simulink model "ArmCast_WrapV2_0"  (Simulink 8.2)
settings: Solver=FixedStepDiscrete  StartTime=0.0  StopTime=Inf  RelTol=1e-3
PreLoadFcn:
  | Ts=0.001;
  | Trajectory = load('CastingTrajectory.mat')
undefined symbols (not defined in the file or in its folder): DiscIntNeverNeededParam
libraries: simulink x15, xpclib x7, speedgoatlib_IO102 x4, speedgoatlib_IO301 x4, xpcutilitieslib x3
(part 1 of 2)
settings Model: Creator=LukePH  LastModifiedBy=LukePH  SimulationMode=external  BufferReuse=off
settings DataIOCC: SignalLoggingSaveFormat=Dataset
settings OptimizationCC: BlockReduction=off  OptimizeBlockIOStorage=off  BufferReuse=off  ExpressionFolding=off  ExpressionDepthLimit=128  LocalBlockOutputs=off
settings DebuggingCC: FcnCallInpInsideContextMsg=EnableAllAsError  StateNameClashWarn=none
settings HardwareCC: ProdIntDivRoundTo=Zero  ProdEndianess=LittleEndian  ProdHWDeviceType=Generic->32-bit x86 compatible
settings RTWCC: SystemTargetFile=xpctarget.tlc  TemplateMakefile=xpc_default_tmf  Description=xPC Target  ProcessScript=xpctarget_make_rtw_hook  RTWCompilerOptimization=On
settings xpcTargetCC: TargetFcnLib=ansi_tfl_table_tmw.mat  CodeReplacementLibrary=XPC_BLAS  ParMdlRefBuildCompliant=on  ConcurrentExecutionCompliant=on  CombineSignalStateStructs=off  MATLABClassNameForMDSCustomization=xpcAperiodicCustomization  GRTInterface=on  GenerateAllocFcn=off  xPCTaskExecutionProfile=off  xPCRL32EventNumber=5000  xPCLoadParamSetFile=off  xPCConcurrentTasks=off  xPCEnableSFAnimation=off

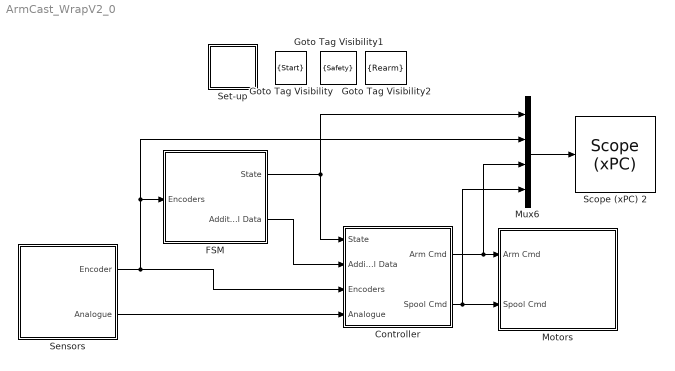
== system ArmCast_WrapV2_0 ==
  Controller : Subsystem
  FSM : Subsystem
  Goto Tag Visibility : GotoTagVisibility  GotoTag=Start
  Goto Tag Visibility1 : GotoTagVisibility  GotoTag=Safety
  Goto Tag Visibility2 : GotoTagVisibility  GotoTag=Rearm
  Motors : Subsystem
  Mux6 : Mux
  Scope (xPC) 2 : xpclib/Misc./Scope (xPC)   scopeno=10  scopetype=File  autostart=on  viewmode=Numerical  formatstr='%15.6f'  grid=on  ylimits=[-2*pi,2*pi]  nosamples=4001  noprepostsamples=0  interleave=4  triggermode=FreeRun  triggersignal=1  trigsignalfromport=off  triggerlevel=0.0  triggerslope=Either  triggerscope=1  triggersample=0  filename=data.dat  mode=Lazy  writesize=512  autorestart=on  dynamicfilemode=off  maxwritefilesize=512*1024^2
  Sensors : Subsystem
  Set-up : Subsystem
  wires:
  Sensors/1(Encoder) -> Controller/3(Encoders), FSM/1(Encoders), Mux6/2
  Sensors/2(Analogue) -> Controller/4(Analogue)
  Controller/1(Arm Cmd) -> Mux6/3, Motors/1(Arm Cmd)
  Controller/2(Spool Cmd) -> Mux6/4, Motors/2(Spool Cmd)
  FSM/1(State) -> Controller/1(State), Mux6/1
  Mux6/1 -> Scope (xPC) 2/1
  FSM/2(Additional Data) -> Controller/2(Additional Data)

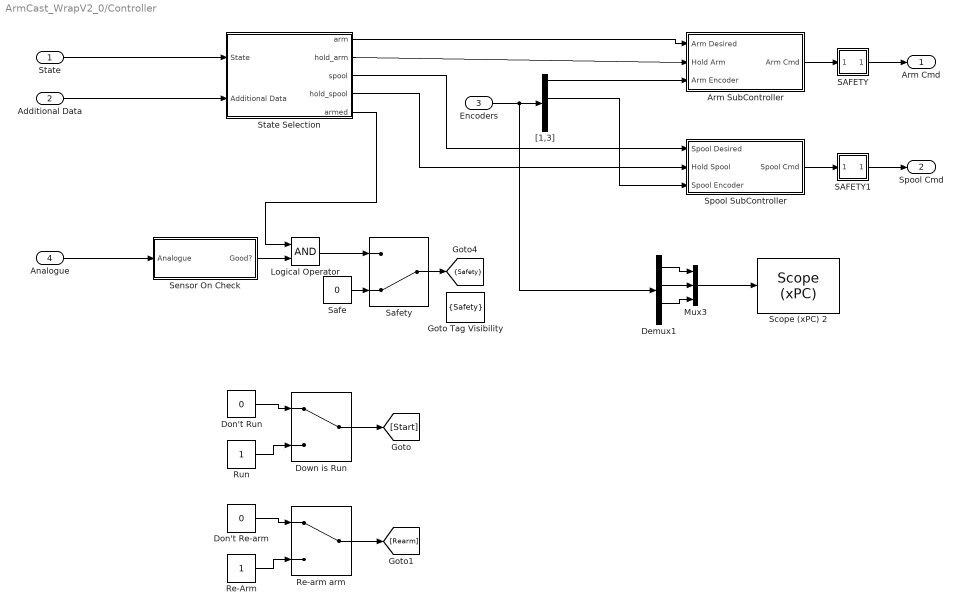
== system ArmCast_WrapV2_0/Controller ==
  State : Inport
  Additional Data : Inport  Port=2
  Encoders : Inport  Port=3
  Analogue : Inport  Port=4
  Arm SubController : Subsystem
  Demux1 : Demux  Outputs=6
  Don't Re-arm : Constant  Value=0
  Don't Run : Constant  Value=0
  Down is Run : ManualSwitch
  Goto Tag Visibility : GotoTagVisibility  GotoTag=Safety
  Logical Operator : Logic  AllPortsSameDT=off  OutDataTypeStr=boolean
  Mux3 : Mux  Inputs=3
  Re-Arm : Constant
  Re-arm arm : ManualSwitch
  Run : Constant
  SAFETY : Subsystem
  SAFETY1 : Subsystem
  Safe : Constant  Value=0
  Safety : ManualSwitch  CurrentSetting=0
  Scope (xPC) 2 : xpclib/Misc./Scope (xPC)   scopeno=4  scopetype=Target  autostart=on  viewmode=Numerical  formatstr='%15.6f'  grid=on  ylimits=[-2*pi,2*pi]  nosamples=250  noprepostsamples=0  interleave=1  triggermode=FreeRun  triggersignal=1  trigsignalfromport=off  triggerlevel=0.0  triggerslope=Either  triggerscope=1  triggersample=0  filename=data.dat  mode=Lazy  writesize=512  autorestart=off  dynamicfilemode=off  maxwritefilesize=512*1024^2
  Sensor On Check : Subsystem
  Spool SubController : Subsystem
  State Selection : Subsystem
  "[1,3]" : Demux  Outputs=6
  Arm Cmd : Outport
  Spool Cmd : Outport  Port=2
  tag scope: Safety=scoped
  wires:
  Safe/1 -> Safety/2
  Safety/1 -> [Safety]
  State Selection/5(armed) -> Logical Operator/1
  State/1 -> State Selection/1(State)
  Encoders/1 -> Demux1/1, "[1,3]"/1
  Analogue/1 -> Sensor On Check/1(Analogue)
  Logical Operator/1 -> Safety/1
  Sensor On Check/1(Good?) -> Logical Operator/2
  Additional Data/1 -> State Selection/2(Additional Data)
  Mux3/1 -> Scope (xPC) 2/1
  Demux1/1 -> Mux3/1
  Demux1/3 -> Mux3/2
  Demux1/5 -> Mux3/3
  State Selection/1(arm) -> Arm SubController/1(Arm Desired)
  "[1,3]"/1 -> Arm SubController/3(Arm Encoder)
  Arm SubController/1(Arm Cmd) -> SAFETY/1(In1)
  SAFETY/1(Out1) -> Arm Cmd/1
  Spool SubController/1(Spool Cmd) -> SAFETY1/1(In1)
  SAFETY1/1(Out1) -> Spool Cmd/1
  State Selection/3(spool) -> Spool SubController/1(Spool Desired)
  State Selection/2(hold_arm) -> Arm SubController/2(Hold Arm)
  State Selection/4(hold_spool) -> Spool SubController/2(Hold Spool)
  "[1,3]"/3 -> Spool SubController/3(Spool Encoder)
  Run/1 -> Down is Run/2
  Don't Run/1 -> Down is Run/1
  Down is Run/1 -> [Start]
  Re-Arm/1 -> Re-arm arm/2
  Don't Re-arm/1 -> Re-arm arm/1
  Re-arm arm/1 -> [Rearm]

== system ArmCast_WrapV2_0/FSM ==
  Encoders : Inport
  Clock : Clock
  Event Handler : Subsystem
  Memory1 : Memory  InheritSampleTime=on
  Switch : Switch  Criteria=u2 > Threshold
  State : Outport
  Additional Data : Outport  Port=2
  wires:
  Switch/1 -> Event Handler/2(Run Start Time), Memory1/1
  Clock/1 -> Switch/3, Event Handler/3(Clock)
  [Start] -> Switch/2, Event Handler/1(Start Signal)
  Memory1/1 -> Switch/1
  Encoders/1 -> Event Handler/4(Encoder)
  [Rearm] -> Event Handler/5(Re-arm)
  Event Handler/1(State) -> State/1
  Event Handler/2(Additional_data) -> Additional Data/1
  [Safety] -> Event Handler/6(Safety)

== system ArmCast_WrapV2_0/Motors ==
  Arm Cmd : Inport
  Spool Cmd : Inport  Port=2
  Analog output : speedgoatlib_IO102/Analog output  id=1  channels=[1,2]  range=1  ts=Ts  pciSlot=-1
  Mux4 : Mux  Inputs=2
  Scope (xPC) 4 : xpclib/Misc./Scope (xPC)   scopeno=6  scopetype=Target  autostart=on  viewmode=Numerical  formatstr='%15.6f'  grid=on  ylimits=[-2*pi,2*pi]  nosamples=250  noprepostsamples=0  interleave=1  triggermode=FreeRun  triggersignal=1  trigsignalfromport=off  triggerlevel=0.0  triggerslope=Either  triggerscope=1  triggersample=0  filename=data.dat  mode=Lazy  writesize=512  autorestart=off  dynamicfilemode=off  maxwritefilesize=512*1024^2
  wires:
  Spool Cmd/1 -> Mux4/2, Analog output/2
  Arm Cmd/1 -> Mux4/1, Analog output/1
  Mux4/1 -> Scope (xPC) 4/1

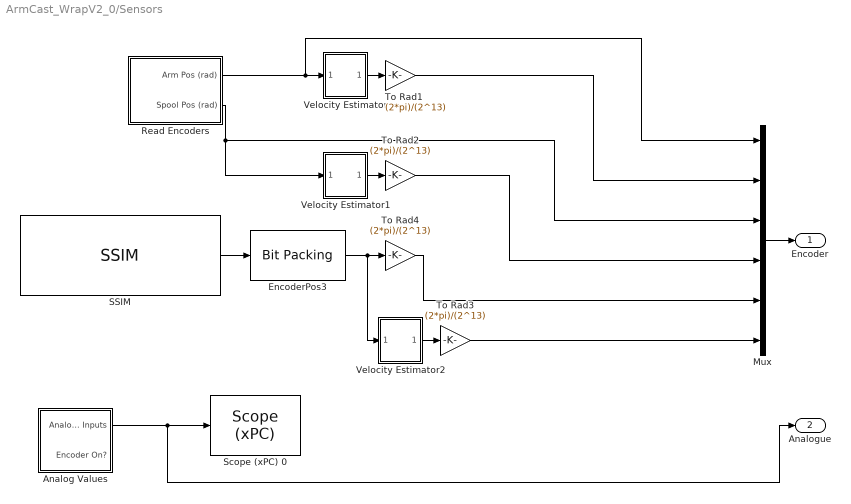
== system ArmCast_WrapV2_0/Sensors ==
  Analog Values : Subsystem
  EncoderPos3 : xpcutilitieslib/Bit Packing   MaskBitPatterns={[0:12]}  MaskPackDataType=int32  MaskPackDataSize=[1]
  Mux : Mux  Inputs=6
  Read Encoders : Subsystem
  SSIM : speedgoatlib_IO301/SSI/SSIM  id=1  chan=[3]  coding=Binary  clockDivider=[200]  wordSize=[13]  TL=[0]  TP=[990]  ssiminv=off  ts=Ts  pciSlot=-1
  "Scope (xPC) 0 " : xpclib/Misc./Scope (xPC)   scopeno=1  scopetype=Target  autostart=on  viewmode=Numerical  formatstr='%15.6f'  grid=on  ylimits=[0,0]  nosamples=250  noprepostsamples=0  interleave=1  triggermode=FreeRun  triggersignal=1  trigsignalfromport=off  triggerlevel=0.0  triggerslope=Either  triggerscope=1  triggersample=0  filename=data.dat  mode=Lazy  writesize=512  autorestart=off  dynamicfilemode=off  maxwritefilesize=512*1024^2
  To Rad{1..4} (4 alike) : Gain  Gain=(2*pi)/(2^13)  OutDataTypeStr=double
  Velocity Estimator : Subsystem  mask{SampleTime=Ts}
      mask prompts: SampleTime "Sample time (-1 for inherited):"
      mask help:
      | This Block takes in encoder values at a rate of 1 sample per Ts seconds and
      | produces an estimate of the velocity at the given time.
      mask TypeOptions SampleTime: Velocity /SystemSampleTime | Weight Calc/SystemSampleTime | Weighted Average/SystemSampleTime | Velocity /Time Constant/Value | Discrete-Time Integrator/SampleTime | Dead Zone/SampleTime | Weight Calc/9000 rad//sec^2 Cut-off/SampleTime | Weight Calc/Discrete Low Pass1/SampleTime | Weight Calc/Discrete Transfer Fcn/SampleTime | Weight Calc/Discrete Transfer Fcn1/SampleTime | Discrete Low Pass2/SampleTime | Velocity /My Difference/Delay/SampleTime | Velocity /My Difference/Sum/SampleTime
      mask Display:
      | port_label('output', 1, '')
      | port_label('input', 1, '')
  Velocity Estimator1 : Subsystem  mask{SampleTime=Ts}
      mask prompts: SampleTime "Sample time (-1 for inherited):"
      mask help:
      | This Block takes in encoder values at a rate of 1 sample per Ts seconds and
      | produces an estimate of the velocity at the given time.
      mask TypeOptions SampleTime: Velocity /SystemSampleTime | Weight Calc/SystemSampleTime | Weighted Average/SystemSampleTime | Velocity /Time Constant/Value | Discrete-Time Integrator/SampleTime | Dead Zone/SampleTime | Weight Calc/9000 rad//sec^2 Cut-off/SampleTime | Weight Calc/Discrete Low Pass1/SampleTime | Weight Calc/Discrete Transfer Fcn/SampleTime | Weight Calc/Discrete Transfer Fcn1/SampleTime | Discrete Low Pass2/SampleTime | Velocity /My Difference/Delay/SampleTime | Velocity /My Difference/Sum/SampleTime
      mask Display:
      | port_label('output', 1, '')
      | port_label('input', 1, '')
  Velocity Estimator2 : Subsystem  mask{SampleTime=Ts}
      mask prompts: SampleTime "Sample time (-1 for inherited):"
      mask help:
      | This Block takes in encoder values at a rate of 1 sample per Ts seconds and
      | produces an estimate of the velocity at the given time.
      mask TypeOptions SampleTime: Velocity /SystemSampleTime | Weight Calc/SystemSampleTime | Weighted Average/SystemSampleTime | Velocity /Time Constant/Value | Discrete-Time Integrator/SampleTime | Dead Zone/SampleTime | Weight Calc/9000 rad//sec^2 Cut-off/SampleTime | Weight Calc/Discrete Low Pass1/SampleTime | Weight Calc/Discrete Transfer Fcn/SampleTime | Weight Calc/Discrete Transfer Fcn1/SampleTime | Discrete Low Pass2/SampleTime | Velocity /My Difference/Delay/SampleTime | Velocity /My Difference/Sum/SampleTime
      mask Display:
      | port_label('output', 1, '')
      | port_label('input', 1, '')
  Encoder : Outport
  Analogue : Outport  Port=2
  wires:
  Velocity Estimator1/1(Out1) -> To Rad2/1
  To Rad1/1 -> Mux/2
  Velocity Estimator/1(Out1) -> To Rad1/1
  Read Encoders/1(Arm Pos (rad)) -> Velocity Estimator/1(In1), Mux/1
  Read Encoders/2(Spool Pos (rad)) -> Velocity Estimator1/1(In1), Mux/3
  SSIM/1 -> EncoderPos3/1
  EncoderPos3/1 -> Velocity Estimator2/1(In1), To Rad4/1
  Velocity Estimator2/1(Out1) -> To Rad3/1
  Mux/1 -> Encoder/1
  To Rad4/1 -> Mux/5
  To Rad3/1 -> Mux/6
  To Rad2/1 -> Mux/4
  Analog Values/1(Analog Inputs) -> Analogue/1, "Scope (xPC) 0 "/1

== system ArmCast_WrapV2_0/Set-up ==
  AnalogSetUp : Subsystem
  Digital output : speedgoatlib_IO301/DIO/Digital output  id=1  channelGroup=Lower  portType=32 ports of type double  lowerDirection=[0,0,0,0,0,0,1,1,1,1,1,1,1,1,1,1]  upperDirection=[1,1,1,1,1,1,1,1,0,0,0,0,0,0,0,0]  ts=Ts  pciSlot=-1
  Disable NST : Constant  Value=0
  Do Not Zero Arm : Constant
  Do Not Zero Spool : Constant
  Setup : speedgoatlib_IO301/Setup/Setup  group=Lower channel group setup  id=1  fpga1=speedgoat_IO301_CI_01230  pciSlot=-1  lowerDirection=[0,0,0,0,0,0,1,1,1,1,1,1,1,1,1,1]  lowerReset=[1]  lowerValue=[1]  upperDirection=[1, 1, 1, 1, 1, 1, 1, 1, 0, 0, 0, 0, 0, 0, 0, 0]  upperReset=[1]  upperValue=[0]
  wires:
  Disable NST/1 -> Digital output/19, Digital output/17
  Do Not Zero Arm/1 -> Digital output/18
  Do Not Zero Spool/1 -> Digital output/20

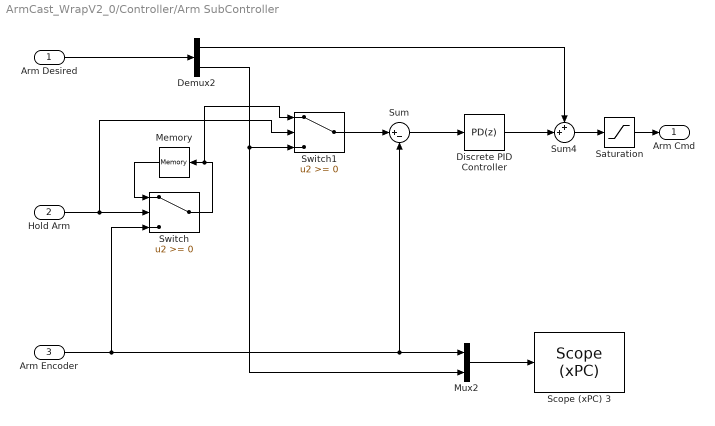
== system ArmCast_WrapV2_0/Controller/Arm SubController ==
  Arm Desired : Inport
  Hold Arm : Inport  Port=2
  Arm Encoder : Inport  Port=3
  Demux2 : Demux  Outputs=2
  Discrete PID Controller : simulink/Continuous/PID Controller  Controller=PD  TimeDomain=Discrete-time  SampleTime=Ts  IntegratorMethod=Forward Euler  FilterMethod=Forward Euler  Form=Parallel  P=30  I=0  D=.15  N=100  InitialConditionSource=internal  InitialConditionForIntegrator=0  InitialConditionForFilter=0  ExternalReset=none  LimitOutput=on  UpperSaturationLimit=6  LowerSaturationLimit=-6  LinearizeAsGain=off  AntiWindupMode=clamping  Kb=1  TrackingMode=off  Kt=1  PParamMin=[]  PParamMax=[]  IParamMin=[]  IParamMax=[]  DParamMin=[]  DParamMax=[]  NParamMin=[]  NParamMax=[]  KbParamMin=[]  KbParamMax=[]  KtParamMin=[]  KtParamMax=[]  POutMin=[]  POutMax=[]  IOutMin=[]  IOutMax=[]  DOutMin=[]  DOutMax=[]  NOutMin=[]  NOutMax=[]  KbOutMin=[]  KbOutMax=[]  KtOutMin=[]  KtOutMax=[]  IntegratorOutMin=[]  IntegratorOutMax=[]  FilterOutMin=[]  FilterOutMax=[]  SumOutMin=[]  SumOutMax=[]  SumI1OutMin=[]  SumI1OutMax=[]  SumI2OutMin=[]  SumI2OutMax=[]  SumI3OutMin=[]  SumI3OutMax=[]  SumDOutMin=[]  SumDOutMax=[]  SaturationOutMin=[]  SaturationOutMax=[]  IntegratorContinuousStateAttributes=''  IntegratorStateMustResolveToSignalObject=off  IntegratorRTWStateStorageClass=Auto  FilterContinuousStateAttributes=''  FilterStateMustResolveToSignalObject=off  FilterRTWStateStorageClass=Auto
  Memory : Memory
  Mux2 : Mux  Inputs=2
  Saturation : Saturate  UpperLimit=6  LowerLimit=-6
  Scope (xPC) 3 : xpclib/Misc./Scope (xPC)   scopeno=2  scopetype=Target  autostart=on  viewmode=Graphical redraw  formatstr='%15.6f'  grid=on  ylimits=[-2*pi,2*pi]  nosamples=250  noprepostsamples=0  interleave=1  triggermode=FreeRun  triggersignal=1  trigsignalfromport=off  triggerlevel=0.0  triggerslope=Either  triggerscope=1  triggersample=0  filename=data.dat  mode=Lazy  writesize=512  autorestart=off  dynamicfilemode=off  maxwritefilesize=512*1024^2
  Sum : Sum  Inputs=|+-
  Sum4 : Sum  Inputs=++|
  Switch : Switch
  Switch1 : Switch
  Arm Cmd : Outport
  wires:
  Mux2/1 -> Scope (xPC) 3/1
  Arm Desired/1 -> Demux2/1
  Sum/1 -> Discrete PID Controller/1
  Saturation/1 -> Arm Cmd/1
  Discrete PID Controller/1 -> Sum4/2
  Sum4/1 -> Saturation/1
  Arm Encoder/1 -> Sum/2, Mux2/1, Switch/3
  Demux2/1 -> Sum4/1
  Demux2/2 -> Switch1/3, Mux2/2
  Switch/1 -> Switch1/1, Memory/1
  Memory/1 -> Switch/1
  Hold Arm/1 -> Switch/2, Switch1/2
  Switch1/1 -> Sum/1

== system ArmCast_WrapV2_0/Controller/SAFETY ==
  In1 : Inport
  Null Cmd2 : Constant  Value=0
  Switch : Switch  Criteria=u2 > Threshold
  Out1 : Outport
  wires:
  Switch/1 -> Out1/1
  Null Cmd2/1 -> Switch/3
  [Safety] -> Switch/2
  In1/1 -> Switch/1

== system ArmCast_WrapV2_0/Controller/SAFETY1 ==
  In1 : Inport
  Null Cmd2 : Constant  Value=0
  Switch : Switch  Criteria=u2 > Threshold
  Out1 : Outport
  wires:
  In1/1 -> Switch/1
  [Safety] -> Switch/2
  Null Cmd2/1 -> Switch/3
  Switch/1 -> Out1/1

== system ArmCast_WrapV2_0/Controller/Sensor On Check ==
  Analogue : Inport
  Constant : Constant  Value=3.25
  Demux1 : Demux
  Relational Operator : RelationalOperator  Operator=>  OutDataTypeStr=fixdt(1,16)
  Good? : Outport
  wires:
  Relational Operator/1 -> Good?/1
  Demux1/4 -> Relational Operator/1
  Constant/1 -> Relational Operator/2
  Analogue/1 -> Demux1/1

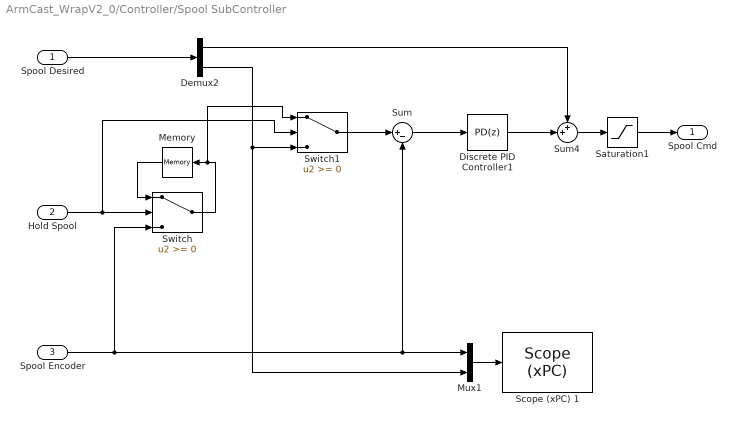
== system ArmCast_WrapV2_0/Controller/Spool SubController ==
  Spool Desired : Inport
  Hold Spool : Inport  Port=2
  Spool Encoder : Inport  Port=3
  Demux2 : Demux  Outputs=2
  Discrete PID Controller1 : simulink/Continuous/PID Controller  Controller=PD  TimeDomain=Discrete-time  SampleTime=Ts  IntegratorMethod=Forward Euler  FilterMethod=Forward Euler  Form=Parallel  P=20  I=0  D=.05  N=100  InitialConditionSource=internal  InitialConditionForIntegrator=0  InitialConditionForFilter=0  ExternalReset=none  LimitOutput=on  UpperSaturationLimit=6  LowerSaturationLimit=-6  LinearizeAsGain=off  AntiWindupMode=clamping  Kb=1  TrackingMode=off  Kt=1  PParamMin=[]  PParamMax=[]  IParamMin=[]  IParamMax=[]  DParamMin=[]  DParamMax=[]  NParamMin=[]  NParamMax=[]  KbParamMin=[]  KbParamMax=[]  KtParamMin=[]  KtParamMax=[]  POutMin=[]  POutMax=[]  IOutMin=[]  IOutMax=[]  DOutMin=[]  DOutMax=[]  NOutMin=[]  NOutMax=[]  KbOutMin=[]  KbOutMax=[]  KtOutMin=[]  KtOutMax=[]  IntegratorOutMin=[]  IntegratorOutMax=[]  FilterOutMin=[]  FilterOutMax=[]  SumOutMin=[]  SumOutMax=[]  SumI1OutMin=[]  SumI1OutMax=[]  SumI2OutMin=[]  SumI2OutMax=[]  SumI3OutMin=[]  SumI3OutMax=[]  SumDOutMin=[]  SumDOutMax=[]  SaturationOutMin=[]  SaturationOutMax=[]  IntegratorContinuousStateAttributes=''  IntegratorStateMustResolveToSignalObject=off  IntegratorRTWStateStorageClass=Auto  FilterContinuousStateAttributes=''  FilterStateMustResolveToSignalObject=off  FilterRTWStateStorageClass=Auto
  Memory : Memory
  Mux1 : Mux  Inputs=2
  Saturation1 : Saturate  UpperLimit=6  LowerLimit=-6
  Scope (xPC) 1 : xpclib/Misc./Scope (xPC)   scopeno=3  scopetype=Target  autostart=on  viewmode=Graphical redraw  formatstr='%15.6f'  grid=on  ylimits=[-2*pi,2*pi]  nosamples=250  noprepostsamples=0  interleave=1  triggermode=FreeRun  triggersignal=1  trigsignalfromport=off  triggerlevel=0.0  triggerslope=Either  triggerscope=1  triggersample=0  filename=data.dat  mode=Lazy  writesize=512  autorestart=off  dynamicfilemode=off  maxwritefilesize=512*1024^2
  Sum : Sum  Inputs=|+-
  Sum4 : Sum  Inputs=++|
  Switch : Switch
  Switch1 : Switch
  Spool Cmd : Outport
  wires:
  Mux1/1 -> Scope (xPC) 1/1
  Saturation1/1 -> Spool Cmd/1
  Spool Desired/1 -> Demux2/1
  Spool Encoder/1 -> Sum/2, Mux1/1, Switch/3
  Demux2/2 -> Switch1/3, Mux1/2
  Switch/1 -> Switch1/1, Memory/1
  Memory/1 -> Switch/1
  Hold Spool/1 -> Switch/2, Switch1/2
  Switch1/1 -> Sum/1
  Sum4/1 -> Saturation1/1
  Discrete PID Controller1/1 -> Sum4/2
  Sum/1 -> Discrete PID Controller1/1
  Demux2/1 -> Sum4/1

== system ArmCast_WrapV2_0/Controller/State Selection ==
  State : Inport
  Additional Data : Inport  Port=2
  Clock2 : Clock
      settings: Decimation=5
  MATLAB Function : MATLAB Function  TreatAsAtomicUnit=on
  Mux : Mux  Inputs=2
  Mux1 : Mux  Inputs=2
  arm : Outport
  hold_arm : Outport  Port=2
  spool : Outport  Port=3
  hold_spool : Outport  Port=4
  armed : Outport  Port=5
  wires:
  Clock2/1 -> MATLAB Function/3(time)
  State/1 -> MATLAB Function/1(state)
  MATLAB Function/7(armed) -> armed/1
  Additional Data/1 -> MATLAB Function/2(additional_data)
  MATLAB Function/3(hold_arm) -> hold_arm/1
  MATLAB Function/6(hold_spool) -> hold_spool/1
  MATLAB Function/1(ud_ar) -> Mux/1
  MATLAB Function/2(xd_ar) -> Mux/2
  Mux/1 -> arm/1
  MATLAB Function/4(ud_sp) -> Mux1/1
  MATLAB Function/5(xd_sp) -> Mux1/2
  Mux1/1 -> spool/1

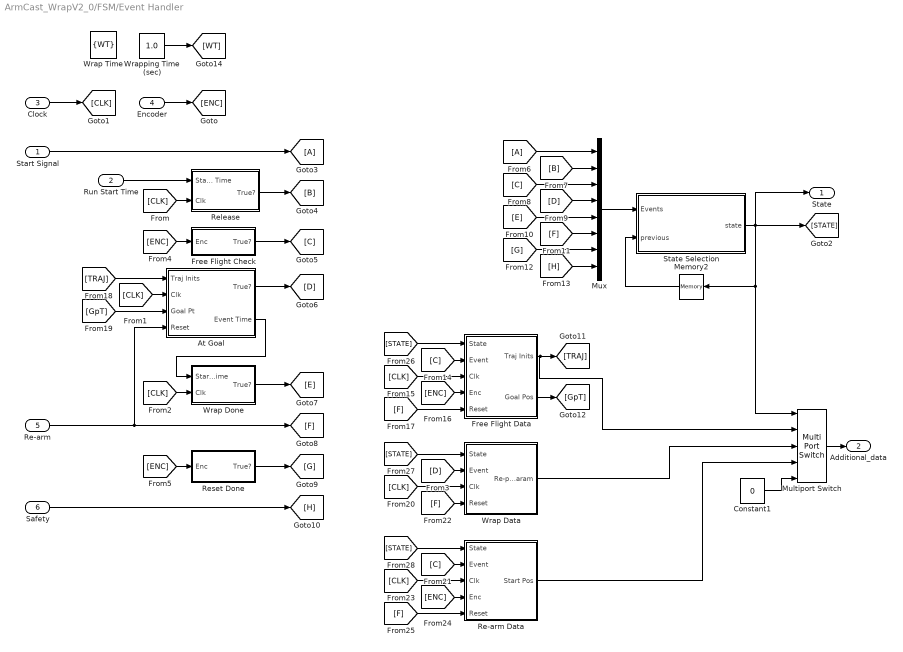
== system ArmCast_WrapV2_0/FSM/Event Handler ==
  Start Signal : Inport
  Run Start Time : Inport  Port=2
  Clock : Inport  Port=3
  Encoder : Inport  Port=4
  Re-arm : Inport  Port=5
  Safety : Inport  Port=6
  At Goal : Subsystem
  Constant1 : Constant  Value=0
  Free Flight Check : Subsystem
  Free Flight Data : Subsystem
  Memory2 : Memory
  Multiport Switch : MultiPortSwitch  Inputs=4
  Mux : Mux  Inputs=8
  Re-arm Data : Subsystem
  Release : Subsystem
  Reset Done : Subsystem
  State Selection : MATLAB Function  TreatAsAtomicUnit=on
  Wrap Data : Subsystem
  Wrap Done : Subsystem
  Wrap Time : GotoTagVisibility  GotoTag=WT
  Wrapping Time (sec) : Constant  Value=1.0
  State : Outport
  Additional_data : Outport  Port=2
  wires:
  Re-arm/1 -> At Goal/4(Reset), [F]
  Run Start Time/1 -> Release/1(Start Time)
  Encoder/1 -> [ENC]
  Clock/1 -> [CLK]
  [CLK] -> Release/2(Clk)
  [CLK] -> At Goal/2(Clk)
  [CLK] -> Wrap Done/2(Clk)
  [ENC] -> Free Flight Check/1(Enc)
  [ENC] -> Reset Done/1(Enc)
  Start Signal/1 -> [A]
  Release/1(True?) -> [B]
  Free Flight Check/1(True?) -> [C]
  At Goal/1(True?) -> [D]
  Wrap Done/1(True?) -> [E]
  Reset Done/1(True?) -> [G]
  Safety/1 -> [H]
  [B] -> Mux/2
  [F] -> Mux/6
  [D] -> Mux/4
  [H] -> Mux/8
  [C] -> Mux/3
  [E] -> Mux/5
  [A] -> Mux/1
  [G] -> Mux/7
  [C] -> Free Flight Data/2(Event)
  [CLK] -> Free Flight Data/3(Clk)
  [ENC] -> Free Flight Data/4(Enc)
  [F] -> Free Flight Data/5(Reset)
  [TRAJ] -> At Goal/1(Traj Inits)
  Free Flight Data/2(Goal Pos) -> [GpT]
  [GpT] -> At Goal/3(Goal Pt)
  At Goal/2(Event Time) -> Wrap Done/1(Start Time)
  [CLK] -> Wrap Data/3(Clk)
  [F] -> Wrap Data/4(Reset)
  Wrap Data/1(Re-pos Param) -> Multiport Switch/3
  Multiport Switch/1 -> Additional_data/1
  Free Flight Data/1(Traj Inits) -> Multiport Switch/2, [TRAJ]
  Wrapping Time (sec)/1 -> [WT]
  [CLK] -> Re-arm Data/3(Clk)
  [ENC] -> Re-arm Data/4(Enc)
  [F] -> Re-arm Data/5(Reset)
  Re-arm Data/1(Start Pos) -> Multiport Switch/4
  Constant1/1 -> Multiport Switch/5
  Mux/1 -> State Selection/1(Events)
  Memory2/1 -> State Selection/2(previous)
  [STATE] -> Free Flight Data/1(State)
  [D] -> Wrap Data/2(Event)
  [STATE] -> Wrap Data/1(State)
  [C] -> Re-arm Data/2(Event)
  [STATE] -> Re-arm Data/1(State)
  State Selection/1(state) -> State/1, [STATE], Multiport Switch/1, Memory2/1

== system ArmCast_WrapV2_0/Sensors/Analog Values ==
  Analog input : speedgoatlib_IO102/Analog input  id=1  channels=[1,2,3,4]  range=1  high_voltage=off  adCoupling=2  ts=Ts  pciSlot=-1
  Constant : Constant  Value=3.25
  Mux : Mux
  Relational Operator : RelationalOperator  Operator=>  OutDataTypeStr=fixdt(1,16)
  Analog Inputs : Outport
  Encoder On? : Outport  Port=2
  wires:
  Mux/1 -> Analog Inputs/1
  Relational Operator/1 -> Encoder On?/1
  Constant/1 -> Relational Operator/2
  Analog input/1 -> Mux/1
  Analog input/2 -> Mux/2
  Analog input/3 -> Mux/3
  Analog input/4 -> Relational Operator/1, Mux/4

== system ArmCast_WrapV2_0/Sensors/Read Encoders ==
  EncoderPos : xpcutilitieslib/Bit Packing   MaskBitPatterns={[0:16]}  MaskPackDataType=int32  MaskPackDataSize=[1]
  EncoderPos1 : xpcutilitieslib/Bit Packing   MaskBitPatterns={[0:16]}  MaskPackDataType=int32  MaskPackDataSize=[1]
  SSIM : speedgoatlib_IO301/SSI/SSIM  id=1  chan=[1:2]  coding=Gray  clockDivider=[200]  wordSize=[17]  TL=[0]  TP=[990]  ssiminv=off  ts=Ts  pciSlot=-1
  Spike Removal : Subsystem
  To Rad : Gain  Gain=(2*pi)/(2^17)  OutDataTypeStr=double
  To Rad1 : Gain  Gain=-(2*pi)/(2^17)  OutDataTypeStr=double
  Wrap Encoder Values : Subsystem
  Arm Pos (rad) : Outport
  Spool Pos (rad) : Outport  Port=2
  wires:
  Wrap Encoder Values/1(Wrapped Values) -> Spike Removal/1(Encoder)
  EncoderPos1/1 -> Wrap Encoder Values/1(Raw Input)
  Spike Removal/1(Filtered) -> To Rad1/1
  To Rad1/1 -> Spool Pos (rad)/1
  SSIM/2 -> EncoderPos1/1
  To Rad/1 -> Arm Pos (rad)/1
  EncoderPos/1 -> To Rad/1
  SSIM/1 -> EncoderPos/1

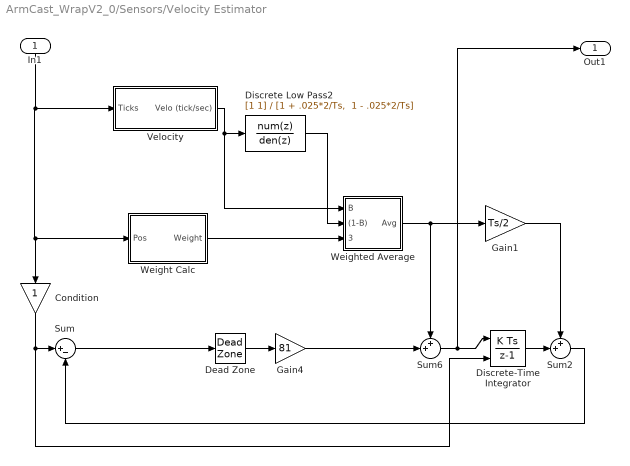
== system ArmCast_WrapV2_0/Sensors/Velocity Estimator ==
  In1 : Inport
  Condition : Gain  OutMin=0  OutMax=10^9  OutDataTypeStr=double
  Dead Zone : DeadZone  LowerValue=-1  UpperValue=1  SampleTime=SampleTime  SaturateOnIntegerOverflow=on
  Discrete Low Pass2 : DiscreteTransferFcn  Numerator=[1 1]  Denominator="[1 + .025*2/Ts,  1 - .025*2/Ts]"  SampleTime=SampleTime
  Discrete-Time Integrator : DiscreteIntegrator  InitialConditionSource=external  SampleTime=SampleTime  ICPrevOutput=DiscIntNeverNeededParam  ICPrevScaledInput=DiscIntNeverNeededParam
  Gain1 : Gain  Gain=Ts/2
  Gain4 : Gain  Gain=81
  Sum : Sum  Inputs=|+-
  Sum2 : Sum  Inputs=++|
  Sum6 : Sum  Inputs=++|
  "Velocity " : Subsystem  SystemSampleTime=SampleTime
  Weight Calc : Subsystem  SystemSampleTime=SampleTime
  Weighted Average : Subsystem  SystemSampleTime=SampleTime
  Out1 : Outport
  wires:
  Condition/1 -> Sum/1, Discrete-Time Integrator/2
  In1/1 -> "Velocity "/1(Ticks), Weight Calc/1(Pos), Condition/1
  "Velocity "/1(Velo (tick/sec)) -> Discrete Low Pass2/1, Weighted Average/1("B ")
  Sum/1 -> Dead Zone/1
  Gain4/1 -> Sum6/2
  Weighted Average/1(Avg) -> Gain1/1, Sum6/1
  Dead Zone/1 -> Gain4/1
  Sum6/1 -> Discrete-Time Integrator/1, Out1/1
  Discrete Low Pass2/1 -> Weighted Average/2((1-B))
  Sum2/1 -> Sum/2
  Discrete-Time Integrator/1 -> Sum2/2
  Gain1/1 -> Sum2/1
  Weight Calc/1(Weight) -> Weighted Average/3(Weight)

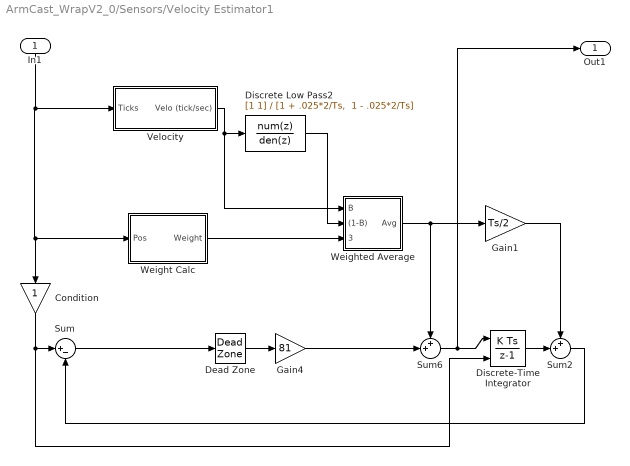
== system ArmCast_WrapV2_0/Sensors/Velocity Estimator1 ==
  In1 : Inport
  Condition : Gain  OutMin=0  OutMax=10^9  OutDataTypeStr=double
  Dead Zone : DeadZone  LowerValue=-1  UpperValue=1  SampleTime=SampleTime  SaturateOnIntegerOverflow=on
  Discrete Low Pass2 : DiscreteTransferFcn  Numerator=[1 1]  Denominator="[1 + .025*2/Ts,  1 - .025*2/Ts]"  SampleTime=SampleTime
  Discrete-Time Integrator : DiscreteIntegrator  InitialConditionSource=external  SampleTime=SampleTime  ICPrevOutput=DiscIntNeverNeededParam  ICPrevScaledInput=DiscIntNeverNeededParam
  Gain1 : Gain  Gain=Ts/2
  Gain4 : Gain  Gain=81
  Sum : Sum  Inputs=|+-
  Sum2 : Sum  Inputs=++|
  Sum6 : Sum  Inputs=++|
  "Velocity " : Subsystem  SystemSampleTime=SampleTime
  Weight Calc : Subsystem  SystemSampleTime=SampleTime
  Weighted Average : Subsystem  SystemSampleTime=SampleTime
  Out1 : Outport
  wires:
  Condition/1 -> Sum/1, Discrete-Time Integrator/2
  In1/1 -> "Velocity "/1(Ticks), Weight Calc/1(Pos), Condition/1
  "Velocity "/1(Velo (tick/sec)) -> Discrete Low Pass2/1, Weighted Average/1("B ")
  Sum/1 -> Dead Zone/1
  Gain4/1 -> Sum6/2
  Weighted Average/1(Avg) -> Gain1/1, Sum6/1
  Dead Zone/1 -> Gain4/1
  Sum6/1 -> Discrete-Time Integrator/1, Out1/1
  Discrete Low Pass2/1 -> Weighted Average/2((1-B))
  Sum2/1 -> Sum/2
  Discrete-Time Integrator/1 -> Sum2/2
  Gain1/1 -> Sum2/1
  Weight Calc/1(Weight) -> Weighted Average/3(Weight)

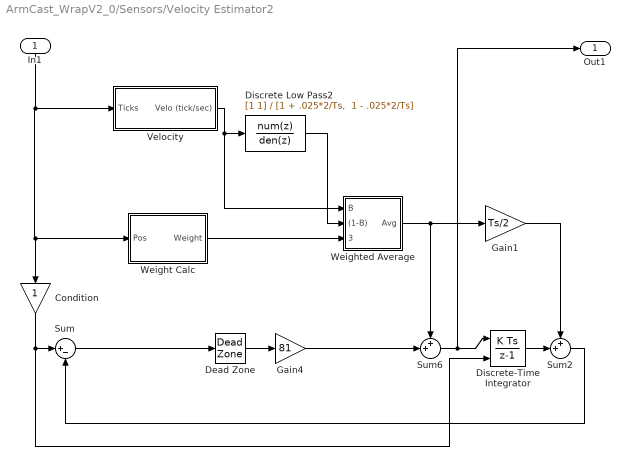
== system ArmCast_WrapV2_0/Sensors/Velocity Estimator2 ==
  In1 : Inport
  Condition : Gain  OutMin=0  OutMax=10^9  OutDataTypeStr=double
  Dead Zone : DeadZone  LowerValue=-1  UpperValue=1  SampleTime=SampleTime  SaturateOnIntegerOverflow=on
  Discrete Low Pass2 : DiscreteTransferFcn  Numerator=[1 1]  Denominator="[1 + .025*2/Ts,  1 - .025*2/Ts]"  SampleTime=SampleTime
  Discrete-Time Integrator : DiscreteIntegrator  InitialConditionSource=external  SampleTime=SampleTime  ICPrevOutput=DiscIntNeverNeededParam  ICPrevScaledInput=DiscIntNeverNeededParam
  Gain1 : Gain  Gain=Ts/2
  Gain4 : Gain  Gain=81
  Sum : Sum  Inputs=|+-
  Sum2 : Sum  Inputs=++|
  Sum6 : Sum  Inputs=++|
  "Velocity " : Subsystem  SystemSampleTime=SampleTime
  Weight Calc : Subsystem  SystemSampleTime=SampleTime
  Weighted Average : Subsystem  SystemSampleTime=SampleTime
  Out1 : Outport
  wires:
  Weight Calc/1(Weight) -> Weighted Average/3(Weight)
  Gain1/1 -> Sum2/1
  Discrete-Time Integrator/1 -> Sum2/2
  Sum2/1 -> Sum/2
  Discrete Low Pass2/1 -> Weighted Average/2((1-B))
  Sum6/1 -> Out1/1, Discrete-Time Integrator/1
  Dead Zone/1 -> Gain4/1
  Weighted Average/1(Avg) -> Sum6/1, Gain1/1
  Gain4/1 -> Sum6/2
  Sum/1 -> Dead Zone/1
  "Velocity "/1(Velo (tick/sec)) -> Weighted Average/1("B "), Discrete Low Pass2/1
  In1/1 -> Condition/1, Weight Calc/1(Pos), "Velocity "/1(Ticks)
  Condition/1 -> Discrete-Time Integrator/2, Sum/1

== system ArmCast_WrapV2_0/Set-up/AnalogSetUp ==
  Analog input : speedgoatlib_IO102/Analog input  Commented=on  id=1  channels=[1,2]  range=1  high_voltage=off  adCoupling=1  ts=Ts  pciSlot=-1
  Mux : Mux  Commented=on  Inputs=2
  Scope (xPC) 1 : xpclib/Misc./Scope (xPC)   Commented=on  scopeno=4  scopetype=Target  autostart=on  viewmode=Graphical redraw  formatstr='%15.6f'  grid=on  ylimits=[0,0]  nosamples=250  noprepostsamples=0  interleave=1  triggermode=FreeRun  triggersignal=1  trigsignalfromport=off  triggerlevel=0.0  triggerslope=Either  triggerscope=1  triggersample=0  filename=data.dat  mode=Lazy  writesize=512  autorestart=off  dynamicfilemode=off  maxwritefilesize=512*1024^2
  SetupAnalog : speedgoatlib_IO102/Setup  group=Analog input setup  id=1  range=+-10V  cal=off  pciSlot=-1  adChannelMode=Multiple-channel (enter number of channels below)  adChannel=4  adCoupling=Single-ended  daChannel=[1,2]  daReset=[1,1]  daInitValue=[0,0]  diChannel=[1]  doChannel=[1]  doReset=[1]  doInitValue=[0]
  wires:
  Mux/1 -> Scope (xPC) 1/1
  Analog input/1 -> Mux/1
  Analog input/2 -> Mux/2

== system ArmCast_WrapV2_0/FSM/Event Handler/At Goal ==
  Traj Inits : Inport
  Clk : Inport  Port=2
  Goal Pt : Inport  Port=3
  Reset : Inport  Port=4
  Latching Switch1 : Subsystem
  MATLAB Function : MATLAB Function  TreatAsAtomicUnit=on
  Memory2 : Memory  X0=false
  True? : Outport
  Event Time : Outport  Port=2
  wires:
  Memory2/1 -> Latching Switch1/2(If True)
  Latching Switch1/1(Out) -> Event Time/1, Memory2/1
  Clk/1 -> MATLAB Function/1(time), Latching Switch1/3(If False)
  Reset/1 -> Latching Switch1/4(Reset)
  Goal Pt/1 -> MATLAB Function/2(goal_pos)
  Traj Inits/1 -> MATLAB Function/3(trajectory_data)
  MATLAB Function/1(True) -> True?/1, Latching Switch1/1(T/F)

== system ArmCast_WrapV2_0/FSM/Event Handler/Free Flight Check ==
  Enc : Inport
  Add : Sum  Inputs=+-
  Compare To Zero : simulink/Logic and Bit Operations/Compare To Zero  relop=>=  OutDataTypeStr=boolean
  Compare To Zero1 : simulink/Logic and Bit Operations/Compare To Zero  relop=>  OutDataTypeStr=boolean
  Demux : Demux  Outputs=6
  Logical Operator : Logic  AllPortsSameDT=off  OutDataTypeStr=boolean
  Memory : Memory
  True? : Outport
  wires:
  Enc/1 -> Demux/1
  Memory/1 -> Add/2
  Add/1 -> Compare To Zero/1
  Compare To Zero1/1 -> Logical Operator/1
  Compare To Zero/1 -> Logical Operator/2
  Logical Operator/1 -> True?/1
  Demux/6 -> Compare To Zero1/1, Add/1, Memory/1

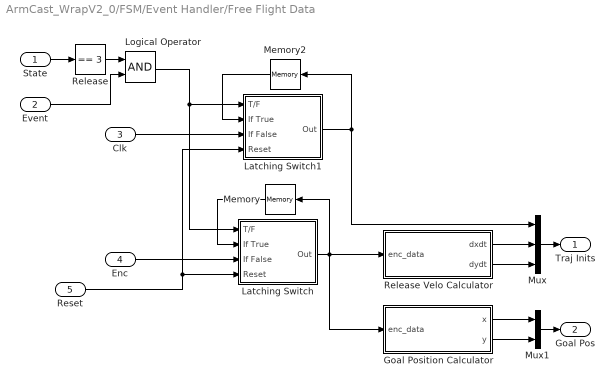
== system ArmCast_WrapV2_0/FSM/Event Handler/Free Flight Data ==
  State : Inport
  Event : Inport  Port=2
  Clk : Inport  Port=3
  Enc : Inport  Port=4
  Reset : Inport  Port=5
  Goal Position Calculator : MATLAB Function  TreatAsAtomicUnit=on
  Latching Switch : Subsystem
  Latching Switch1 : Subsystem
  Logical Operator : Logic  AllPortsSameDT=off  OutDataTypeStr=boolean
  Memory : Memory  X0=false
  Memory2 : Memory  X0=false
  Mux : Mux  Inputs=3
  Mux1 : Mux  Inputs=2
  Release : simulink/Logic and Bit Operations/Compare To Constant  relop===  const=3  OutDataTypeStr=boolean
  Release Velo Calculator : MATLAB Function  TreatAsAtomicUnit=on
  Traj Inits : Outport
  Goal Pos : Outport  Port=2
  wires:
  Event/1 -> Logical Operator/2
  Latching Switch/1(Out) -> Goal Position Calculator/1(enc_data), Memory/1, Release Velo Calculator/1(enc_data)
  Memory/1 -> Latching Switch/2(If True)
  Release Velo Calculator/1(dxdt) -> Mux/2
  Release Velo Calculator/2(dydt) -> Mux/3
  Latching Switch1/1(Out) -> Memory2/1, Mux/1
  Reset/1 -> Latching Switch1/4(Reset), Latching Switch/4(Reset)
  Memory2/1 -> Latching Switch1/2(If True)
  Clk/1 -> Latching Switch1/3(If False)
  Mux/1 -> Traj Inits/1
  Enc/1 -> Latching Switch/3(If False)
  Goal Position Calculator/2(y) -> Mux1/2
  Goal Position Calculator/1(x) -> Mux1/1
  Mux1/1 -> Goal Pos/1
  State/1 -> Release/1
  Release/1 -> Logical Operator/1
  Logical Operator/1 -> Latching Switch/1(T/F), Latching Switch1/1(T/F)

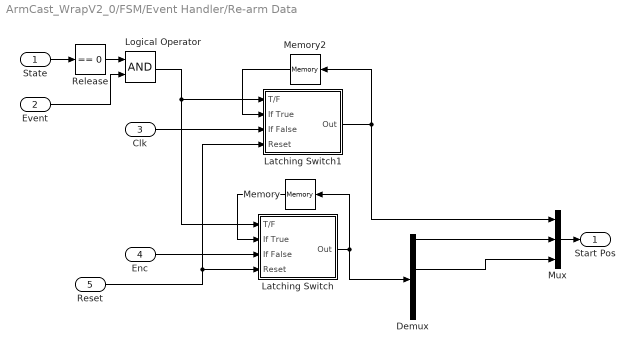
== system ArmCast_WrapV2_0/FSM/Event Handler/Re-arm Data ==
  State : Inport
  Event : Inport  Port=2
  Clk : Inport  Port=3
  Enc : Inport  Port=4
  Reset : Inport  Port=5
  Demux : Demux  Outputs=6
  Latching Switch : Subsystem
  Latching Switch1 : Subsystem
  Logical Operator : Logic  AllPortsSameDT=off  OutDataTypeStr=boolean
  Memory : Memory  X0=false
  Memory2 : Memory  X0=false
  Mux : Mux  Inputs=3
  Release : simulink/Logic and Bit Operations/Compare To Constant  relop===  const=0  OutDataTypeStr=boolean
  Start Pos : Outport
  wires:
  Enc/1 -> Latching Switch/3(If False)
  Mux/1 -> Start Pos/1
  Clk/1 -> Latching Switch1/3(If False)
  Memory2/1 -> Latching Switch1/2(If True)
  Reset/1 -> Latching Switch/4(Reset), Latching Switch1/4(Reset)
  Latching Switch1/1(Out) -> Mux/1, Memory2/1
  Memory/1 -> Latching Switch/2(If True)
  Latching Switch/1(Out) -> Memory/1, Demux/1
  Logical Operator/1 -> Latching Switch/1(T/F), Latching Switch1/1(T/F)
  Demux/1 -> Mux/2
  Demux/3 -> Mux/3
  Event/1 -> Logical Operator/2
  State/1 -> Release/1
  Release/1 -> Logical Operator/1

== system ArmCast_WrapV2_0/FSM/Event Handler/Release ==
  Start Time : Inport
  Clk : Inport  Port=2
  Add1 : Sum  Inputs=+-
  Relational Operator : RelationalOperator  OutDataTypeStr=boolean
  Release Time : Constant  Value=2.6
  True? : Outport
  wires:
  Start Time/1 -> Add1/2
  Relational Operator/1 -> True?/1
  Clk/1 -> Add1/1
  Release Time/1 -> Relational Operator/2
  Add1/1 -> Relational Operator/1

== system ArmCast_WrapV2_0/FSM/Event Handler/Reset Done ==
  Enc : Inport
  Abs : Abs
  Arm : Sum  Inputs=+-
  Compare To Constant : simulink/Logic and Bit Operations/Compare To Constant  relop=<  const=.1  OutDataTypeStr=boolean
  Compare To Constant1 : simulink/Logic and Bit Operations/Compare To Constant  relop=<  const=.2  OutDataTypeStr=boolean
  Constant : Constant  Value=pi
  Demux : Demux  Outputs=6
  Logical Operator : Logic  AllPortsSameDT=off  OutDataTypeStr=boolean
  Spool : Abs
  True? : Outport
  wires:
  Enc/1 -> Demux/1
  Demux/1 -> Arm/1
  Constant/1 -> Arm/2
  Arm/1 -> Abs/1
  Demux/3 -> Spool/1
  Abs/1 -> Compare To Constant/1
  Spool/1 -> Compare To Constant1/1
  Compare To Constant/1 -> Logical Operator/1
  Compare To Constant1/1 -> Logical Operator/2
  Logical Operator/1 -> True?/1

== system ArmCast_WrapV2_0/FSM/Event Handler/Wrap Data ==
  State : Inport
  Event : Inport  Port=2
  Clk : Inport  Port=3
  Reset : Inport  Port=4
  Arm Angle Rate (Rad/sec) : Constant  Value=.5
  Latching Switch1 : Subsystem
  Logical Operator : Logic  AllPortsSameDT=off  OutDataTypeStr=boolean
  Memory2 : Memory  X0=false
  Mux : Mux  Inputs=3
  Release : simulink/Logic and Bit Operations/Compare To Constant  relop===  const=4  OutDataTypeStr=boolean
  Sum : Sum  Inputs=++|
  Re-pos Param : Outport
  wires:
  Mux/1 -> Re-pos Param/1
  Clk/1 -> Latching Switch1/3(If False)
  Memory2/1 -> Latching Switch1/2(If True)
  Reset/1 -> Latching Switch1/4(Reset)
  Latching Switch1/1(Out) -> Sum/1, Mux/1, Memory2/1
  [WT] -> Sum/2
  Sum/1 -> Mux/2
  Arm Angle Rate (Rad/sec)/1 -> Mux/3
  Event/1 -> Logical Operator/2
  State/1 -> Release/1
  Release/1 -> Logical Operator/1
  Logical Operator/1 -> Latching Switch1/1(T/F)

== system ArmCast_WrapV2_0/FSM/Event Handler/Wrap Done ==
  Start Time : Inport
  Clk : Inport  Port=2
  Add1 : Sum  Inputs=+-
  Relational Operator : RelationalOperator  OutDataTypeStr=boolean
  True? : Outport
  wires:
  [WT] -> Relational Operator/2
  Add1/1 -> Relational Operator/1
  Clk/1 -> Add1/1
  Start Time/1 -> Add1/2
  Relational Operator/1 -> True?/1

== system ArmCast_WrapV2_0/Sensors/Read Encoders/Spike Removal ==
  Encoder : Inport
  Abs1 : Abs
  Delay1 : Delay  DelayLength=1  InitialCondition=0  SampleTime=Ts
  Memory1 : Memory  InheritSampleTime=on
  Relational Operator2 : RelationalOperator  OutDataTypeStr=boolean
  Spike height : Constant  Value=130000
  Sum2 : Sum  Inputs=|-+
  Switch2 : Switch  Criteria=u2 > Threshold  SampleTime=Ts
  Filtered : Outport
  wires:
  Relational Operator2/1 -> Switch2/2
  Sum2/1 -> Abs1/1
  Spike height/1 -> Relational Operator2/2
  Abs1/1 -> Relational Operator2/1
  Encoder/1 -> Delay1/1, Switch2/3, Sum2/2
  Memory1/1 -> Switch2/1
  Delay1/1 -> Sum2/1
  Switch2/1 -> Memory1/1, Filtered/1

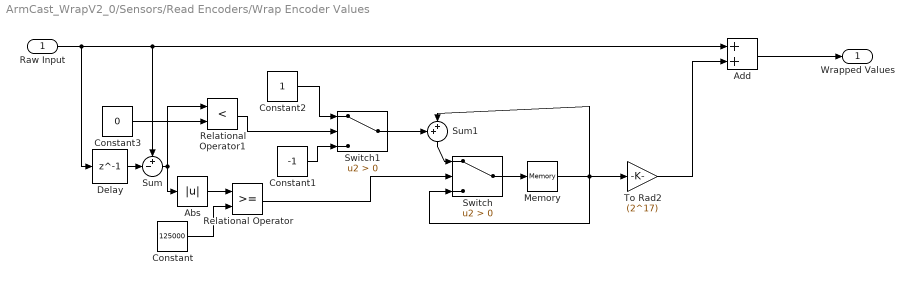
== system ArmCast_WrapV2_0/Sensors/Read Encoders/Wrap Encoder Values ==
  Raw Input : Inport
  Abs : Abs
  Add : Sum
  Constant : Constant  Value=125000
  Constant1 : Constant  Value=-1
  Constant2 : Constant
  Constant3 : Constant  Value=0
  Delay : Delay  DelayLength=1  InitialCondition=0  SampleTime=Ts
  Memory : Memory  InheritSampleTime=on
  Relational Operator : RelationalOperator  OutDataTypeStr=boolean
  Relational Operator1 : RelationalOperator  Operator=<  OutDataTypeStr=boolean
  Sum : Sum  Inputs=+-|
  Sum1 : Sum  Inputs=++|
  Switch : Switch  Criteria=u2 > Threshold  SampleTime=Ts
  Switch1 : Switch  Criteria=u2 > Threshold  SampleTime=Ts
  To Rad2 : Gain  Gain=(2^17)  OutDataTypeStr=double
  Wrapped Values : Outport
  wires:
  To Rad2/1 -> Add/2
  Constant3/1 -> Relational Operator1/2
  Abs/1 -> Relational Operator/1
  Sum/1 -> Abs/1, Relational Operator1/1
  Constant2/1 -> Switch1/1
  Relational Operator1/1 -> Switch1/2
  Constant1/1 -> Switch1/3
  Switch1/1 -> Sum1/1
  Memory/1 -> To Rad2/1, Switch/3, Sum1/2
  Switch/1 -> Memory/1
  Delay/1 -> Sum/2
  Sum1/1 -> Switch/1
  Relational Operator/1 -> Switch/2
  Constant/1 -> Relational Operator/2
  Add/1 -> Wrapped Values/1
  Raw Input/1 -> Add/1, Sum/1, Delay/1

== system ArmCast_WrapV2_0/Sensors/Velocity Estimator/Velocity  ==
  Ticks : Inport  SampleTime=Ts
  Divide : Product  Inputs=*/
  Memory : Memory
  Memory1 : Memory  X0=Ts
  Memory2 : Memory
  My Difference : Subsystem
  Sum1 : Sum  Inputs=|++
  Switch : Switch  Criteria=u2 ~= 0
  Switch1 : Switch  Criteria=u2 ~= 0
  Switch2 : Switch  Criteria=u2 ~= 0
  Time Constant : Constant  Value=SampleTime
  Velo (tick/sec) : Outport  SampleTime=Ts
  wires:
  Switch2/1 -> Memory2/1, Velo (tick/sec)/1
  Memory2/1 -> Switch2/3
  Divide/1 -> Switch2/1
  Memory1/1 -> Divide/2, Sum1/2
  Sum1/1 -> Switch1/3
  Time Constant/1 -> Sum1/1, Switch1/1
  Switch1/1 -> Memory1/1
  Memory/1 -> Switch/3
  Switch/1 -> Memory/1, Divide/1
  My Difference/1(Out1) -> Switch/2, Switch2/2, Switch1/2, Switch/1
  Ticks/1 -> My Difference/1(In1)

== system ArmCast_WrapV2_0/Sensors/Velocity Estimator/Weight Calc ==
  Pos : Inport
  29731 rad/sec^2 Cut-off : Saturate  UpperLimit=29731  LowerLimit=0  SampleTime=SampleTime
  Abs : Abs  OutMin=0  OutMax=10^9  OutDataTypeStr=fixdt(1,16)
  Difference : simulink/Discrete/Difference  ICPrevInput=0.0  InputProcessing=Inherited  OutMin=[]  OutMax=[]  OutDataType=fixdt(1, 16)  OutScaling=2^-10  DoSatur=off
  Difference1 : simulink/Discrete/Difference  ICPrevInput=0.0  InputProcessing=Inherited  OutMin=[]  OutMax=[]  OutDataType=fixdt(1, 16)  OutScaling=2^-10  DoSatur=off
  Discrete Low Pass1 : DiscreteTransferFcn  Numerator=[1 1]  Denominator="[1 + .5*2/Ts,  1 - .5*2/Ts]"  SampleTime=SampleTime
  Discrete Transfer Fcn : DiscreteTransferFcn  Numerator=[1 0]  Denominator="[.015 + Ts/2,  -.015 + Ts/2]"  SampleTime=SampleTime
  Discrete Transfer Fcn1 : DiscreteTransferFcn  Numerator=[1 0]  Denominator="[.15 + Ts/2,  -.15 + Ts/2]"  SampleTime=SampleTime
  Gain : Gain  Gain=1/29731
  Weight : Outport  SampleTime=Ts
  wires:
  Discrete Low Pass1/1 -> 29731 rad/sec^2 Cut-off/1
  Abs/1 -> Discrete Low Pass1/1
  Discrete Transfer Fcn/1 -> Abs/1
  Pos/1 -> Difference1/1
  Discrete Transfer Fcn1/1 -> Difference/1
  Difference/1 -> Discrete Transfer Fcn/1
  Difference1/1 -> Discrete Transfer Fcn1/1
  29731 rad/sec^2 Cut-off/1 -> Gain/1
  Gain/1 -> Weight/1

== system ArmCast_WrapV2_0/Sensors/Velocity Estimator/Weighted Average ==
  "B " : Inport
  (1-B) : Inport  Port=2
  Weight : Inport  Port=3
  Constant : Constant
  Product : Product  RndMeth=Zero
  Product1 : Product  RndMeth=Zero
  Sum : Sum  Inputs=+-|
  Sum1 : Sum  Inputs=++|
  Avg : Outport
  wires:
  Sum1/1 -> Avg/1
  Product/1 -> Sum1/1
  Product1/1 -> Sum1/2
  Sum/1 -> Product1/1
  Constant/1 -> Sum/1
  (1-B)/1 -> Product1/2
  Weight/1 -> Sum/2, Product/1
  "B "/1 -> Product/2

== system ArmCast_WrapV2_0/Sensors/Velocity Estimator1/Velocity  ==
  Ticks : Inport  SampleTime=Ts
  Divide : Product  Inputs=*/
  Memory : Memory
  Memory1 : Memory  X0=Ts
  Memory2 : Memory
  My Difference : Subsystem
  Sum1 : Sum  Inputs=|++
  Switch : Switch  Criteria=u2 ~= 0
  Switch1 : Switch  Criteria=u2 ~= 0
  Switch2 : Switch  Criteria=u2 ~= 0
  Time Constant : Constant  Value=SampleTime
  Velo (tick/sec) : Outport  SampleTime=Ts
  wires:
  Switch2/1 -> Memory2/1, Velo (tick/sec)/1
  Memory2/1 -> Switch2/3
  Divide/1 -> Switch2/1
  Memory1/1 -> Divide/2, Sum1/2
  Sum1/1 -> Switch1/3
  Time Constant/1 -> Sum1/1, Switch1/1
  Switch1/1 -> Memory1/1
  Memory/1 -> Switch/3
  Switch/1 -> Memory/1, Divide/1
  My Difference/1(Out1) -> Switch/2, Switch2/2, Switch1/2, Switch/1
  Ticks/1 -> My Difference/1(In1)

== system ArmCast_WrapV2_0/Sensors/Velocity Estimator1/Weight Calc ==
  Pos : Inport
  29731 rad/sec^2 Cut-off : Saturate  UpperLimit=29731  LowerLimit=0  SampleTime=SampleTime
  Abs : Abs  OutMin=0  OutMax=10^9  OutDataTypeStr=fixdt(1,16)
  Difference : simulink/Discrete/Difference  ICPrevInput=0.0  InputProcessing=Inherited  OutMin=[]  OutMax=[]  OutDataType=fixdt(1, 16)  OutScaling=2^-10  DoSatur=off
  Difference1 : simulink/Discrete/Difference  ICPrevInput=0.0  InputProcessing=Inherited  OutMin=[]  OutMax=[]  OutDataType=fixdt(1, 16)  OutScaling=2^-10  DoSatur=off
  Discrete Low Pass1 : DiscreteTransferFcn  Numerator=[1 1]  Denominator="[1 + .5*2/Ts,  1 - .5*2/Ts]"  SampleTime=SampleTime
  Discrete Transfer Fcn : DiscreteTransferFcn  Numerator=[1 0]  Denominator="[.015 + Ts/2,  -.015 + Ts/2]"  SampleTime=SampleTime
  Discrete Transfer Fcn1 : DiscreteTransferFcn  Numerator=[1 0]  Denominator="[.15 + Ts/2,  -.15 + Ts/2]"  SampleTime=SampleTime
  Gain : Gain  Gain=1/29731
  Weight : Outport  SampleTime=Ts
  wires:
  Discrete Low Pass1/1 -> 29731 rad/sec^2 Cut-off/1
  Abs/1 -> Discrete Low Pass1/1
  Discrete Transfer Fcn/1 -> Abs/1
  Pos/1 -> Difference1/1
  Discrete Transfer Fcn1/1 -> Difference/1
  Difference/1 -> Discrete Transfer Fcn/1
  Difference1/1 -> Discrete Transfer Fcn1/1
  29731 rad/sec^2 Cut-off/1 -> Gain/1
  Gain/1 -> Weight/1

== system ArmCast_WrapV2_0/Sensors/Velocity Estimator1/Weighted Average ==
  "B " : Inport
  (1-B) : Inport  Port=2
  Weight : Inport  Port=3
  Constant : Constant
  Product : Product  RndMeth=Zero
  Product1 : Product  RndMeth=Zero
  Sum : Sum  Inputs=+-|
  Sum1 : Sum  Inputs=++|
  Avg : Outport
  wires:
  Sum1/1 -> Avg/1
  Product/1 -> Sum1/1
  Product1/1 -> Sum1/2
  Sum/1 -> Product1/1
  Constant/1 -> Sum/1
  (1-B)/1 -> Product1/2
  Weight/1 -> Sum/2, Product/1
  "B "/1 -> Product/2

== system ArmCast_WrapV2_0/Sensors/Velocity Estimator2/Velocity  ==
  Ticks : Inport  SampleTime=Ts
  Divide : Product  Inputs=*/
  Memory : Memory
  Memory1 : Memory  X0=Ts
  Memory2 : Memory
  My Difference : Subsystem
  Sum1 : Sum  Inputs=|++
  Switch : Switch  Criteria=u2 ~= 0
  Switch1 : Switch  Criteria=u2 ~= 0
  Switch2 : Switch  Criteria=u2 ~= 0
  Time Constant : Constant  Value=SampleTime
  Velo (tick/sec) : Outport  SampleTime=Ts
  wires:
  Ticks/1 -> My Difference/1(In1)
  My Difference/1(Out1) -> Switch/1, Switch1/2, Switch2/2, Switch/2
  Switch/1 -> Divide/1, Memory/1
  Memory/1 -> Switch/3
  Switch1/1 -> Memory1/1
  Time Constant/1 -> Switch1/1, Sum1/1
  Sum1/1 -> Switch1/3
  Memory1/1 -> Sum1/2, Divide/2
  Divide/1 -> Switch2/1
  Memory2/1 -> Switch2/3
  Switch2/1 -> Velo (tick/sec)/1, Memory2/1

== system ArmCast_WrapV2_0/Sensors/Velocity Estimator2/Weight Calc ==
  Pos : Inport
  29731 rad/sec^2 Cut-off : Saturate  UpperLimit=29731  LowerLimit=0  SampleTime=SampleTime
  Abs : Abs  OutMin=0  OutMax=10^9  OutDataTypeStr=fixdt(1,16)
  Difference : simulink/Discrete/Difference  ICPrevInput=0.0  InputProcessing=Inherited  OutMin=[]  OutMax=[]  OutDataType=fixdt(1, 16)  OutScaling=2^-10  DoSatur=off
  Difference1 : simulink/Discrete/Difference  ICPrevInput=0.0  InputProcessing=Inherited  OutMin=[]  OutMax=[]  OutDataType=fixdt(1, 16)  OutScaling=2^-10  DoSatur=off
  Discrete Low Pass1 : DiscreteTransferFcn  Numerator=[1 1]  Denominator="[1 + .5*2/Ts,  1 - .5*2/Ts]"  SampleTime=SampleTime
  Discrete Transfer Fcn : DiscreteTransferFcn  Numerator=[1 0]  Denominator="[.015 + Ts/2,  -.015 + Ts/2]"  SampleTime=SampleTime
  Discrete Transfer Fcn1 : DiscreteTransferFcn  Numerator=[1 0]  Denominator="[.15 + Ts/2,  -.15 + Ts/2]"  SampleTime=SampleTime
  Gain : Gain  Gain=1/29731
  Weight : Outport  SampleTime=Ts
  wires:
  Gain/1 -> Weight/1
  29731 rad/sec^2 Cut-off/1 -> Gain/1
  Difference1/1 -> Discrete Transfer Fcn1/1
  Difference/1 -> Discrete Transfer Fcn/1
  Discrete Transfer Fcn1/1 -> Difference/1
  Pos/1 -> Difference1/1
  Discrete Transfer Fcn/1 -> Abs/1
  Abs/1 -> Discrete Low Pass1/1
  Discrete Low Pass1/1 -> 29731 rad/sec^2 Cut-off/1

== system ArmCast_WrapV2_0/Sensors/Velocity Estimator2/Weighted Average ==
  "B " : Inport
  (1-B) : Inport  Port=2
  Weight : Inport  Port=3
  Constant : Constant
  Product : Product  RndMeth=Zero
  Product1 : Product  RndMeth=Zero
  Sum : Sum  Inputs=+-|
  Sum1 : Sum  Inputs=++|
  Avg : Outport
  wires:
  "B "/1 -> Product/2
  Weight/1 -> Product/1, Sum/2
  (1-B)/1 -> Product1/2
  Constant/1 -> Sum/1
  Sum/1 -> Product1/1
  Product1/1 -> Sum1/2
  Product/1 -> Sum1/1
  Sum1/1 -> Avg/1

== system ArmCast_WrapV2_0/FSM/Event Handler/At Goal/Latching Switch1 ==
  T/F : Inport
  If True : Inport  Port=2
  If False : Inport  Port=3
  Reset : Inport  Port=4
  Constant1 : Constant  Value=true
  Constant2 : Constant  Value=false
  Logical Operator : Logic  Operator=OR  AllPortsSameDT=off  OutDataTypeStr=boolean
  Memory : Memory  X0=false
  Switch : Switch
  Switch1 : Switch
  Switch2 : Switch
  Out : Outport
  wires:
  Memory/1 -> Switch/3
  Logical Operator/1 -> Switch1/2
  T/F/1 -> Switch/2, Logical Operator/2
  Switch2/1 -> Memory/1, Logical Operator/1
  If True/1 -> Switch1/1
  Switch/1 -> Switch2/3
  Switch1/1 -> Out/1
  Constant1/1 -> Switch/1
  Reset/1 -> Switch2/2
  If False/1 -> Switch1/3
  Constant2/1 -> Switch2/1

== system ArmCast_WrapV2_0/FSM/Event Handler/Free Flight Data/Latching Switch ==
  T/F : Inport
  If True : Inport  Port=2
  If False : Inport  Port=3
  Reset : Inport  Port=4
  Constant1 : Constant  Value=true
  Constant2 : Constant  Value=false
  Logical Operator : Logic  Operator=OR  AllPortsSameDT=off  OutDataTypeStr=boolean
  Memory : Memory  X0=false
  Switch : Switch
  Switch1 : Switch
  Switch2 : Switch
  Out : Outport
  wires:
  Memory/1 -> Switch/3
  Logical Operator/1 -> Switch1/2
  T/F/1 -> Switch/2, Logical Operator/2
  Switch2/1 -> Memory/1, Logical Operator/1
  If True/1 -> Switch1/1
  Switch/1 -> Switch2/3
  Switch1/1 -> Out/1
  Constant1/1 -> Switch/1
  Reset/1 -> Switch2/2
  If False/1 -> Switch1/3
  Constant2/1 -> Switch2/1

== system ArmCast_WrapV2_0/FSM/Event Handler/Free Flight Data/Latching Switch1 ==
  T/F : Inport
  If True : Inport  Port=2
  If False : Inport  Port=3
  Reset : Inport  Port=4
  Constant1 : Constant  Value=true
  Constant2 : Constant  Value=false
  Logical Operator : Logic  Operator=OR  AllPortsSameDT=off  OutDataTypeStr=boolean
  Memory : Memory  X0=false
  Switch : Switch
  Switch1 : Switch
  Switch2 : Switch
  Out : Outport
  wires:
  Memory/1 -> Switch/3
  Logical Operator/1 -> Switch1/2
  T/F/1 -> Switch/2, Logical Operator/2
  Switch2/1 -> Memory/1, Logical Operator/1
  If True/1 -> Switch1/1
  Switch/1 -> Switch2/3
  Switch1/1 -> Out/1
  Constant1/1 -> Switch/1
  Reset/1 -> Switch2/2
  If False/1 -> Switch1/3
  Constant2/1 -> Switch2/1

== system ArmCast_WrapV2_0/FSM/Event Handler/Re-arm Data/Latching Switch ==
  T/F : Inport
  If True : Inport  Port=2
  If False : Inport  Port=3
  Reset : Inport  Port=4
  Constant1 : Constant  Value=true
  Constant2 : Constant  Value=false
  Logical Operator : Logic  Operator=OR  AllPortsSameDT=off  OutDataTypeStr=boolean
  Memory : Memory  X0=false
  Switch : Switch
  Switch1 : Switch
  Switch2 : Switch
  Out : Outport
  wires:
  Constant2/1 -> Switch2/1
  If False/1 -> Switch1/3
  Reset/1 -> Switch2/2
  Constant1/1 -> Switch/1
  Switch1/1 -> Out/1
  Switch/1 -> Switch2/3
  If True/1 -> Switch1/1
  Switch2/1 -> Logical Operator/1, Memory/1
  T/F/1 -> Logical Operator/2, Switch/2
  Logical Operator/1 -> Switch1/2
  Memory/1 -> Switch/3

== system ArmCast_WrapV2_0/FSM/Event Handler/Re-arm Data/Latching Switch1 ==
  T/F : Inport
  If True : Inport  Port=2
  If False : Inport  Port=3
  Reset : Inport  Port=4
  Constant1 : Constant  Value=true
  Constant2 : Constant  Value=false
  Logical Operator : Logic  Operator=OR  AllPortsSameDT=off  OutDataTypeStr=boolean
  Memory : Memory  X0=false
  Switch : Switch
  Switch1 : Switch
  Switch2 : Switch
  Out : Outport
  wires:
  Constant2/1 -> Switch2/1
  If False/1 -> Switch1/3
  Reset/1 -> Switch2/2
  Constant1/1 -> Switch/1
  Switch1/1 -> Out/1
  Switch/1 -> Switch2/3
  If True/1 -> Switch1/1
  Switch2/1 -> Logical Operator/1, Memory/1
  T/F/1 -> Logical Operator/2, Switch/2
  Logical Operator/1 -> Switch1/2
  Memory/1 -> Switch/3

== system ArmCast_WrapV2_0/FSM/Event Handler/Wrap Data/Latching Switch1 ==
  T/F : Inport
  If True : Inport  Port=2
  If False : Inport  Port=3
  Reset : Inport  Port=4
  Constant1 : Constant  Value=true
  Constant2 : Constant  Value=false
  Logical Operator : Logic  Operator=OR  AllPortsSameDT=off  OutDataTypeStr=boolean
  Memory : Memory  X0=false
  Switch : Switch
  Switch1 : Switch
  Switch2 : Switch
  Out : Outport
  wires:
  Constant2/1 -> Switch2/1
  If False/1 -> Switch1/3
  Reset/1 -> Switch2/2
  Constant1/1 -> Switch/1
  Switch1/1 -> Out/1
  Switch/1 -> Switch2/3
  If True/1 -> Switch1/1
  Switch2/1 -> Logical Operator/1, Memory/1
  T/F/1 -> Logical Operator/2, Switch/2
  Logical Operator/1 -> Switch1/2
  Memory/1 -> Switch/3

== system ArmCast_WrapV2_0/Sensors/Velocity Estimator/Velocity /My Difference ==
  In1 : Inport
  Delay : Delay  DelayLength=1  InitialConditionSource=Input port  SampleTime=Ts
      settings: InputPortMap=u0,p4
  Sum : Sum  Inputs=|+-  SampleTime=Ts
  Out1 : Outport
  wires:
  Delay/1 -> Sum/2
  Sum/1 -> Out1/1
  In1/1 -> Delay/1, Sum/1, Delay/2

== system ArmCast_WrapV2_0/Sensors/Velocity Estimator1/Velocity /My Difference ==
  In1 : Inport
  Delay : Delay  DelayLength=1  InitialConditionSource=Input port  SampleTime=Ts
      settings: InputPortMap=u0,p4
  Sum : Sum  Inputs=|+-  SampleTime=Ts
  Out1 : Outport
  wires:
  Delay/1 -> Sum/2
  Sum/1 -> Out1/1
  In1/1 -> Delay/1, Sum/1, Delay/2

== system ArmCast_WrapV2_0/Sensors/Velocity Estimator2/Velocity /My Difference ==
  In1 : Inport
  Delay : Delay  DelayLength=1  InitialConditionSource=Input port  SampleTime=Ts
      settings: InputPortMap=u0,p4
  Sum : Sum  Inputs=|+-  SampleTime=Ts
  Out1 : Outport
  wires:
  In1/1 -> Delay/2, Sum/1, Delay/1
  Sum/1 -> Out1/1
  Delay/1 -> Sum/2
